simulink model "torque_control_z"  (R2023b)
settings: Solver=FixedStepAuto  StartTime=0.0  StopTime=10  RelTol=1e-3  EnableMultiTasking=on
undefined symbols (not defined in the file): G_v
libraries: cstblocks x3
settings Model: ExtModeTrigDuration=10  Creator=miche  LastModifiedBy=miche
settings OptimizationCC: EnhancedBackFolding=on  PassReuseOutputArgsAs=Individual arguments  ZeroExternalMemoryAtStartup=off  ZeroInternalMemoryAtStartup=off  MaxStackSize=64  OptimizeBlockOrder=speed  DifferentSizesBufferReuse=on  OptimizationCustomize=off  EfficientTunableParamExpr=on
settings DebuggingCC: ParameterTunabilityLossMsg=error
settings HardwareCC: ProdBitPerPointer=32  ProdBitPerSizeT=32  ProdBitPerPtrDiffT=32  ProdLargestAtomicInteger=Long  ProdLargestAtomicFloat=Double  ProdWordSize=32  ProdLongLongMode=on  ProdHWDeviceType=ARM Compatible->ARM Cortex
settings SFSimCC: MATLABDynamicMemAlloc=off
settings RTWCC: Description=Embedded Coder  SystemTargetFile=ert.tlc  HardwareBoard=STM32 Nucleo F401RE  TemplateMakefile=ert_default_tmf  Toolchain=GNU Tools for ARM Embedded Processors  PortableWordSizes=on
settings CodeAppCC: ForceParamTrailComments=on  IgnoreCustomStorageClasses=off  OperatorAnnotations=on  SimulinkDataObjDesc=on  SFDataObjDesc=on  InsertBlockDesc=on
settings ERTTargetCC: ExtModeTransport=3  ExtModeStaticAlloc=on  ExtModeStaticAllocSize=2000  ExtModeMexFile=ext_xcp  ExtModeIntrfLevel=Level2 - Open

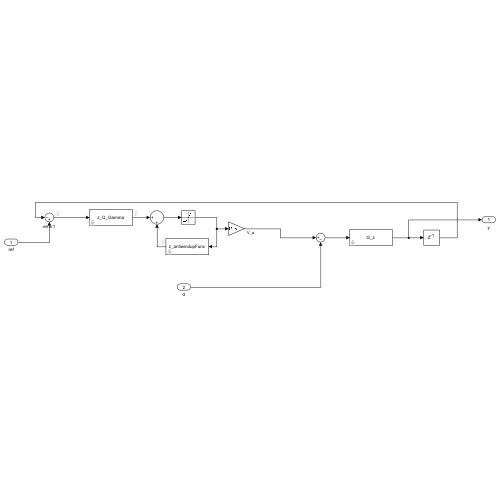
[thumbnail: Simulink's stored preview of the top-level diagram]
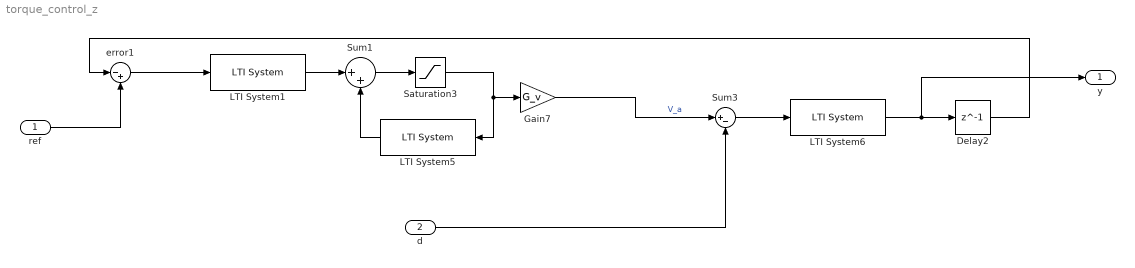
== system torque_control_z ==
  ref : Inport  OutDataTypeStr=double  PortDimensions=1  Interpolate=off
  d : Inport  Port=2  OutDataTypeStr=double  PortDimensions=1  Interpolate=off
  Delay2 : Delay  DelayLength=1
  Gain7 : Gain  Gain=G_v
  LTI System1 : cstblocks/LTI System  sys=z_Q_Gamma  IC=[]  PadeOrder=0
  LTI System5 : cstblocks/LTI System  sys=z_antiwindupFunc  IC=[]  PadeOrder=0
  LTI System6 : cstblocks/LTI System  sys=G_z  IC=[]  PadeOrder=0
  Saturation3 : Saturate  UpperLimit=12  LowerLimit=-12
  Sum1 : Sum  Inputs=|++
  Sum3 : Sum  Inputs=|+-
  error1 : Sum  Inputs=|-+
  y : Outport  OutDataTypeStr=double  VectorParamsAs1DForOutWhenUnconnected=off
  wires:
  Saturation3/1 -> Gain7/1, LTI System5/1
  Delay2/1 -> error1/1
  Sum3/1 -> LTI System6/1
  LTI System6/1 -> y/1, Delay2/1
  LTI System5/1 -> Sum1/2
  LTI System1/1 -> Sum1/1
  error1/1 -> LTI System1/1
  Sum1/1 -> Saturation3/1
  Gain7/1 -> Sum3/1  "V_a"
  d/1 -> Sum3/2
  ref/1 -> error1/2
